simulink model "fuzzy_pi_simulink"  (R2013a)
settings: Solver=ode23tb  StartTime=0.0  StopTime=300  RelTol=1e-3
libraries: fuzblock x1, simulink x1
settings Model: Creator=paulo.costa  LastModifiedBy=paulo.costa

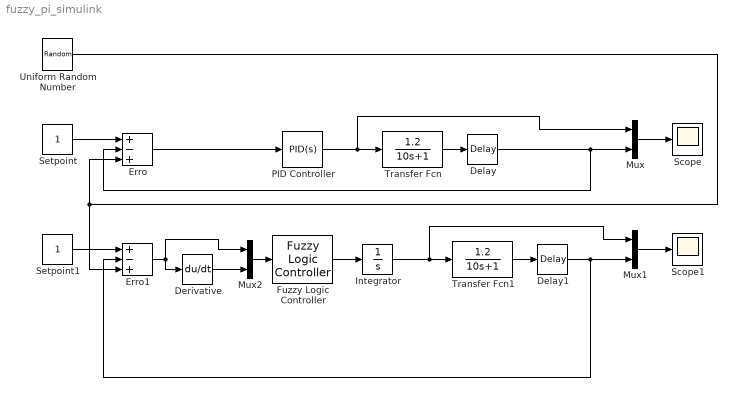
== system fuzzy_pi_simulink ==
  Delay : TransportDelay  DelayTime=2
  Delay1 : TransportDelay  DelayTime=2
  Derivative : Derivative
  Erro : Sum  Inputs=+-+
  Erro1 : Sum  Inputs=+-+
  Fuzzy Logic Controller : fuzblock/Fuzzy Logic  Controller  fis=fuzzy_pi
  Integrator : Integrator
  Mux : Mux  Inputs=2
  Mux1 : Mux  Inputs=2
  Mux2 : Mux  Inputs=2
  PID Controller : simulink/Continuous/PID Controller  Controller=PID  TimeDomain=Continuous-time  SampleTime=1  IntegratorMethod=Forward Euler  FilterMethod=Forward Euler  Form=Parallel  P=3  I=1.25  D=0  N=100  InitialConditionSource=internal  InitialConditionForIntegrator=0  InitialConditionForFilter=0  ExternalReset=none  LimitOutput=off  UpperSaturationLimit=inf  LowerSaturationLimit=-inf  LinearizeAsGain=on  AntiWindupMode=none  Kb=1  TrackingMode=off  Kt=1  PParamMin=[]  PParamMax=[]  IParamMin=[]  IParamMax=[]  DParamMin=[]  DParamMax=[]  NParamMin=[]  NParamMax=[]  KbParamMin=[]  KbParamMax=[]  KtParamMin=[]  KtParamMax=[]  POutMin=[]  POutMax=[]  IOutMin=[]  IOutMax=[]  DOutMin=[]  DOutMax=[]  NOutMin=[]  NOutMax=[]  KbOutMin=[]  KbOutMax=[]  KtOutMin=[]  KtOutMax=[]  IntegratorOutMin=[]  IntegratorOutMax=[]  FilterOutMin=[]  FilterOutMax=[]  SumOutMin=[]  SumOutMax=[]  SumI1OutMin=[]  SumI1OutMax=[]  SumI2OutMin=[]  SumI2OutMax=[]  SumI3OutMin=[]  SumI3OutMax=[]  SumDOutMin=[]  SumDOutMax=[]  SaturationOutMin=[]  SaturationOutMax=[]  IntegratorContinuousStateAttributes=''  IntegratorStateMustResolveToSignalObject=off  IntegratorRTWStateStorageClass=Auto  FilterContinuousStateAttributes=''  FilterStateMustResolveToSignalObject=off  FilterRTWStateStorageClass=Auto
  Scope : Scope
  Scope1 : Scope
  Setpoint : Constant
  Setpoint1 : Constant
  Transfer Fcn : TransferFcn  Numerator=[1.2]  Denominator=[10 1]
  Transfer Fcn1 : TransferFcn  Numerator=[1.2]  Denominator=[10 1]
  Uniform Random Number : UniformRandomNumber  Minimum=-.1  Maximum=.1  SampleTime=0.1
  wires:
  Transfer Fcn/1 -> Delay/1
  PID Controller/1 -> Mux/1, Transfer Fcn/1
  Erro/1 -> PID Controller/1
  Setpoint/1 -> Erro/1
  Delay/1 -> Mux/2, Erro/2
  Mux/1 -> Scope/1
  Transfer Fcn1/1 -> Delay1/1
  Setpoint1/1 -> Erro1/1
  Delay1/1 -> Mux1/2, Erro1/2
  Mux1/1 -> Scope1/1
  Fuzzy Logic Controller/1 -> Integrator/1
  Erro1/1 -> Derivative/1, Mux2/1
  Mux2/1 -> Fuzzy Logic Controller/1
  Derivative/1 -> Mux2/2
  Integrator/1 -> Mux1/1, Transfer Fcn1/1
  Uniform Random Number/1 -> Erro/3, Erro1/3
